simulink model "model"  (R2021b)
settings: Solver=VariableStepAuto  StartTime=0.0  StopTime=10.0  RelTol=1e-3
undefined symbols (not defined in the file): DiscIntNeverNeededParam
libraries: simulink x3, slpidlib x2
settings Model: Creator=O  LastModifiedBy=wangzixuan

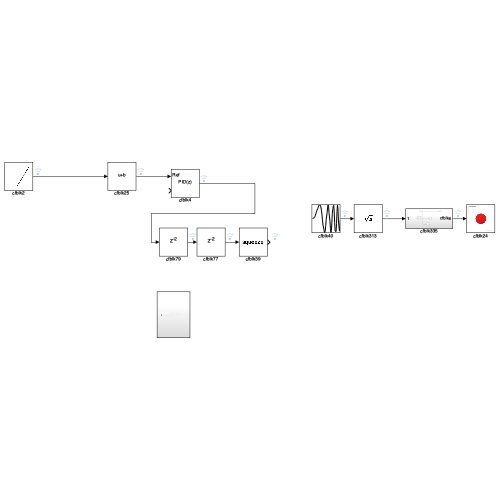
[thumbnail: Simulink's stored preview of the top-level diagram]
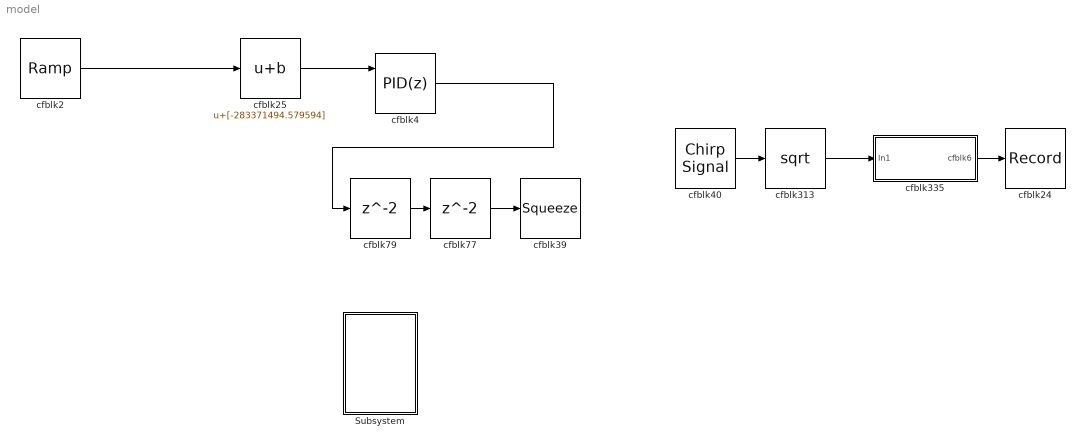
== system model ==
  Subsystem : Subsystem
  cfblk2 : simulink/Sources/Ramp  slope=[3073.754164]  start=[6.066803]  InitialOutput=[561595.891675]
  cfblk24 : Record  FileSettingsInternal="{\"entries\":[{\"content\":{\"excelSettings\":{\"content\":{},\"type\":\"Streamout.ExcelSettings\"}},\"type\":\"Streamout.FileSettingStorage\",\"uuid\":\"9c569ba5-3f76-45be-a7ff-ea8434ca4ceb\"}],\"packageUris\":[\"http://schema.mathworks.com/mf0/streamout_blocks/R2020a\"],\"version\":\"1.0\"}"  SignalsInternal="{\"entries\":[{\"content\":{\"signals\":[{\"content\":{\"blockPath\":[\"model/cfblk24\"],\"channel\":[],\"dimensions\":[1],\"domain\":\"model/cfblk24\",\"lineColor\":\"#ff13a6\",\"plots\":[1],\"port\":1,\"sid\":[],\"signalID\":585911,\"signalName\":\"cfblk335\"},\"type\":\"RecordBlkView.Signal\",\"uuid\":\"b2ada7c7-cfb3-4a8e-b65c-6ed73041aef6\"}]},\"type\":\"RecordBlkView.InputSignals\",\"uuid\":\"04f6ddc4-06cc-4646-89bd-e82fc14adc66\"}],\"packageUris\":[\"http://schema.mathworks.com/mf0/streamout_blocks/R2020a\"],\"version\":\"1.0\"}"  VisualizationBindings="{\"sparklinesplugin\":{\"info\":[{\"bindingParametersList\":[],\"subplotID\":1}]}}"
  cfblk25 : Bias  Bias=[-283371494.579594]
  cfblk313 : Sqrt  OutDataTypeStr=double  SaturateOnIntegerOverflow=on
  cfblk335 : Subsystem
  cfblk39 : Squeeze
  cfblk4 : slpidlib/PID Controller (2DOF)  Controller=PID  Form=Parallel  TimeDomain=Discrete-time  UseExternalTs=off  SampleTime=1  IntegratorMethod=Forward Euler  FilterMethod=Forward Euler  ControllerParametersSource=internal  P=1  I=1  D=0  UseFilter=on  N=100  b=1  c=1  TunerSelectOption=Transfer Function Based (PID Tuner App)  InitialConditionSource=internal  InitialConditionForIntegrator=0  InitialConditionForFilter=0  DifferentiatorICPrevScaledInput=0  ExternalReset=none  TrackingMode=off  Kt=1  LimitOutput=off  SatLimitsSource=internal  UpperSaturationLimit=inf  LowerSaturationLimit=-inf  LinearizeAsGain=off  AntiWindupMode=none  Kb=1  POutMin=[]  POutMax=[]  IOutMin=[]  IOutMax=[]  DOutMin=[]  DOutMax=[]  NOutMin=[]  NOutMax=[]  bOutMin=[]  bOutMax=[]  cOutMin=[]  cOutMax=[]  SumOutMin=[]  SumOutMax=[]  SaturationOutMin=[]  SaturationOutMax=[]  PParamMin=[]  PParamMax=[]  IParamMin=[]  IParamMax=[]  DParamMin=[]  DParamMax=[]  NParamMin=[]  NParamMax=[]  bParamMin=[]  bParamMax=[]  cParamMin=[]  cParamMax=[]  KbParamMin=[]  KbParamMax=[]  KtParamMin=[]  KtParamMax=[]  KbOutMin=[]  KbOutMax=[]  KtOutMin=[]  KtOutMax=[]  IntegratorOutMin=[]  IntegratorOutMax=[]  FilterOutMin=[]  FilterOutMax=[]  SumI1OutMin=[]  SumI1OutMax=[]  SumI2OutMin=[]  SumI2OutMax=[]  SumI3OutMin=[]  SumI3OutMax=[]  SumI4OutMin=[]  SumI4OutMax=[]  SumDOutMin=[]  SumDOutMax=[]  Sum1OutMin=[]  Sum1OutMax=[]  Sum2OutMin=[]  Sum2OutMax=[]  Sum3OutMin=[]  Sum3OutMax=[]  DifferentiatorOutMin=[]  DifferentiatorOutMax=[]  FilterDiffOutCoefMin=[]  FilterDiffOutCoefMax=[]  ReciprocalOutMin=[]  ReciprocalOutMax=[]  SumDenOutMin=[]  SumDenOutMax=[]  SumNumOutMin=[]  SumNumOutMax=[]  DivideOutMin=[]  DivideOutMax=[]  UdiffTsProdOutMin=[]  UdiffTsProdOutMax=[]  NTsProdOutMin=[]  NTsProdOutMax=[]  UintegralTsProdOutMin=[]  UintegralTsProdOutMax=[]  UngainTsProdOutMin=[]  UngainTsProdOutMax=[]  IntegratorContinuousStateAttributes=''  IntegratorStateMustResolveToSignalObject=off  IntegratorRTWStateStorageClass=Auto  FilterContinuousStateAttributes=''  FilterStateMustResolveToSignalObject=off  FilterRTWStateStorageClass=Auto  ParallelPVariant=InternalParameters  IdealPVariant=Disabled  IVariant=InternalParameters  DVariant=InternalParameters  bVariant=InternalParameters  cVariant=InternalParameters  IntegratorVariant=Discrete  SatVariant=Disabled  AWVariant=Passthrough  PCopyVariant=Disabled  TRVariant=Disabled  FdbkBlocksVariant=Forward  IdealPFdbkVariant=Disabled  SatFdbkVariant=Disabled  DerivativeFilterVariant=ForwardEulerFilter  NVariant=InternalParameters  NCopyVariant=Disabled  FilterICVariant=InternalICsFilter  IntegratorICVariant=InternalICs  ExternalResetVariant=Disabled  TRSumVariant=Passthrough  SumFdbkVariant=Disabled  SumVariant=Sum_PID  TsampFilterVariant=InternalTs  TsampNgainVariant=Passthrough  TsampIntegralVariant=Passthrough  ExternalSaturationOutDataTypeStr=Inherit: Same as second input
      settings: SourceProductBaseCode=SL
  cfblk40 : simulink/Sources/Chirp Signal  f1=[890112838.698821]  T=[783698053.297768]  f2=[819425252.339437]
  cfblk77 : Delay  SampleTime=1
  cfblk79 : Delay  SampleTime=1
  wires:
  cfblk335/1(cfblk6) -> cfblk24/1
  cfblk313/1 -> cfblk335/1(In1)
  cfblk40/1 -> cfblk313/1
  cfblk77/1 -> cfblk39/1
  cfblk2/1 -> cfblk25/1
  cfblk79/1 -> cfblk77/1
  cfblk4/1 -> cfblk79/1
  cfblk25/1 -> cfblk4/1

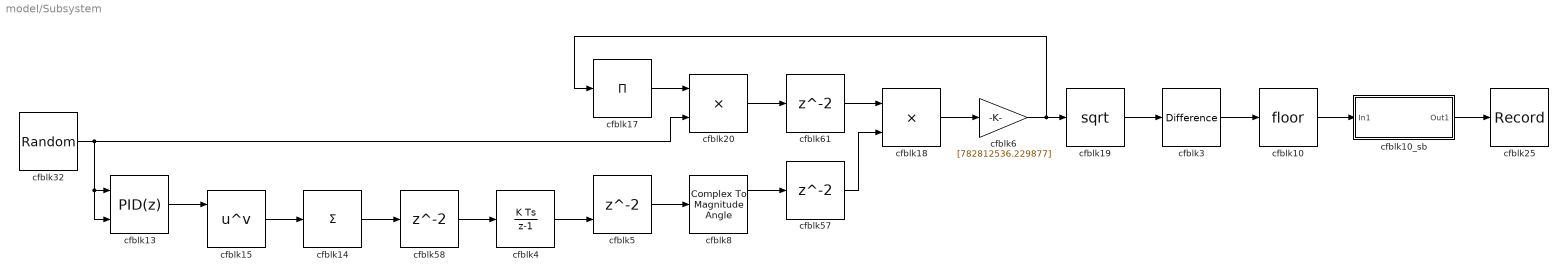
== system model/Subsystem ==
  cfblk10 : Rounding
  cfblk10_sb : Subsystem
  cfblk13 : slpidlib/PID Controller (2DOF)  Controller=PID  Form=Parallel  TimeDomain=Discrete-time  UseExternalTs=off  SampleTime=1  IntegratorMethod=Forward Euler  FilterMethod=Forward Euler  ControllerParametersSource=internal  P=1  I=1  D=0  UseFilter=on  N=100  b=1  c=1  TunerSelectOption=Transfer Function Based (PID Tuner App)  InitialConditionSource=internal  InitialConditionForIntegrator=0  InitialConditionForFilter=0  DifferentiatorICPrevScaledInput=0  ExternalReset=none  TrackingMode=off  Kt=1  LimitOutput=off  SatLimitsSource=internal  UpperSaturationLimit=inf  LowerSaturationLimit=-inf  LinearizeAsGain=off  AntiWindupMode=none  Kb=1  POutMin=[]  POutMax=[]  IOutMin=[]  IOutMax=[]  DOutMin=[]  DOutMax=[]  NOutMin=[]  NOutMax=[]  bOutMin=[]  bOutMax=[]  cOutMin=[]  cOutMax=[]  SumOutMin=[]  SumOutMax=[]  SaturationOutMin=[]  SaturationOutMax=[]  PParamMin=[]  PParamMax=[]  IParamMin=[]  IParamMax=[]  DParamMin=[]  DParamMax=[]  NParamMin=[]  NParamMax=[]  bParamMin=[]  bParamMax=[]  cParamMin=[]  cParamMax=[]  KbParamMin=[]  KbParamMax=[]  KtParamMin=[]  KtParamMax=[]  KbOutMin=[]  KbOutMax=[]  KtOutMin=[]  KtOutMax=[]  IntegratorOutMin=[]  IntegratorOutMax=[]  FilterOutMin=[]  FilterOutMax=[]  SumI1OutMin=[]  SumI1OutMax=[]  SumI2OutMin=[]  SumI2OutMax=[]  SumI3OutMin=[]  SumI3OutMax=[]  SumI4OutMin=[]  SumI4OutMax=[]  SumDOutMin=[]  SumDOutMax=[]  Sum1OutMin=[]  Sum1OutMax=[]  Sum2OutMin=[]  Sum2OutMax=[]  Sum3OutMin=[]  Sum3OutMax=[]  DifferentiatorOutMin=[]  DifferentiatorOutMax=[]  FilterDiffOutCoefMin=[]  FilterDiffOutCoefMax=[]  ReciprocalOutMin=[]  ReciprocalOutMax=[]  SumDenOutMin=[]  SumDenOutMax=[]  SumNumOutMin=[]  SumNumOutMax=[]  DivideOutMin=[]  DivideOutMax=[]  UdiffTsProdOutMin=[]  UdiffTsProdOutMax=[]  NTsProdOutMin=[]  NTsProdOutMax=[]  UintegralTsProdOutMin=[]  UintegralTsProdOutMax=[]  UngainTsProdOutMin=[]  UngainTsProdOutMax=[]  IntegratorContinuousStateAttributes=''  IntegratorStateMustResolveToSignalObject=off  IntegratorRTWStateStorageClass=Auto  FilterContinuousStateAttributes=''  FilterStateMustResolveToSignalObject=off  FilterRTWStateStorageClass=Auto  ParallelPVariant=InternalParameters  IdealPVariant=Disabled  IVariant=InternalParameters  DVariant=InternalParameters  bVariant=InternalParameters  cVariant=InternalParameters  IntegratorVariant=Discrete  SatVariant=Disabled  AWVariant=Passthrough  PCopyVariant=Disabled  TRVariant=Disabled  FdbkBlocksVariant=Forward  IdealPFdbkVariant=Disabled  SatFdbkVariant=Disabled  DerivativeFilterVariant=ForwardEulerFilter  NVariant=InternalParameters  NCopyVariant=Disabled  FilterICVariant=InternalICsFilter  IntegratorICVariant=InternalICs  ExternalResetVariant=Disabled  TRSumVariant=Passthrough  SumFdbkVariant=Disabled  SumVariant=Sum_PID  TsampFilterVariant=InternalTs  TsampNgainVariant=Passthrough  TsampIntegralVariant=Passthrough  ExternalSaturationOutDataTypeStr=Inherit: Same as second input
      settings: SourceProductBaseCode=SL
  cfblk14 : Sum  Inputs=+  OutDataTypeStr=double
  cfblk15 : Math  Operator=pow  OutDataTypeStr=double  SaturateOnIntegerOverflow=on
  cfblk17 : Product  Inputs=*  OutDataTypeStr=double
  cfblk18 : Product  Inputs=**  OutDataTypeStr=double
  cfblk19 : Sqrt  OutDataTypeStr=double  SaturateOnIntegerOverflow=on
  cfblk20 : Product  Inputs=**  OutDataTypeStr=double
  cfblk25 : Record  FileSettingsInternal="{\"entries\":[{\"content\":{\"excelSettings\":{\"content\":{},\"type\":\"Streamout.ExcelSettings\"}},\"type\":\"Streamout.FileSettingStorage\",\"uuid\":\"7687e2ec-381f-4673-acb7-97b648be0800\"}],\"packageUris\":[\"http://schema.mathworks.com/mf0/streamout_blocks/R2020a\"],\"version\":\"1.0\"}"  SignalsInternal="{\"entries\":[{\"content\":{\"signals\":[{\"content\":{\"blockPath\":[\"model/Subsystem/cfblk25\"],\"channel\":[],\"dimensions\":[1],\"domain\":\"model/Subsystem/cfblk25\",\"lineColor\":\"#d95319\",\"plots\":[1],\"port\":1,\"sid\":[],\"signalID\":585916,\"signalName\":\"cfblk10_sb\"},\"type\":\"RecordBlkView.Signal\",\"uuid\":\"a16bbc3b-36d9-44fd-905f-6b673a140423\"}]},\"type\":\"RecordBlkView.InputSignals\",\"uuid\":\"f5bc2cff-cab3-458f-b6f2-1f37294e6b90\"}],\"packageUris\":[\"http://schema.mathworks.com/mf0/streamout_blocks/R2020a\"],\"version\":\"1.0\"}"  VisualizationBindings="{\"sparklinesplugin\":{\"info\":[{\"bindingParametersList\":[],\"subplotID\":1}]}}"
  cfblk3 : simulink/Discrete/Difference  ICPrevInput=0.0  OutMin=[]  OutMax=[]  OutDataTypeStr=double  OutputDataTypeScalingMode=double  OutDataType=fixdt(1, 16)  OutScaling=2^-10  DoSatur=off
  cfblk32 : RandomNumber  Mean=[-73598.078492]  Variance=[73248.164035]  Seed=[877060262.000000]  SampleTime=0.1
  cfblk4 : DiscreteIntegrator  OutDataTypeStr=double  ICPrevOutput=DiscIntNeverNeededParam  ICPrevScaledInput=DiscIntNeverNeededParam
  cfblk5 : Delay  ShowEnablePort=on  SampleTime=1
      settings: InputPortMap=u0,e6
  cfblk57 : Delay  SampleTime=1
  cfblk58 : Delay  SampleTime=1
  cfblk6 : Gain  Gain=[782812536.229877]  OutDataTypeStr=double
  cfblk61 : Delay  SampleTime=1
  cfblk8 : ComplexToMagnitudeAngle
  wires:
  cfblk19/1 -> cfblk3/1
  cfblk57/1 -> cfblk18/2
  cfblk14/1 -> cfblk58/1
  cfblk6/1 -> cfblk19/1, cfblk17/1
  cfblk10_sb/1(Out1) -> cfblk25/1
  cfblk13/1 -> cfblk15/1
  cfblk18/1 -> cfblk6/1
  cfblk15/1 -> cfblk14/1
  cfblk20/1 -> cfblk61/1
  cfblk3/1 -> cfblk10/1
  cfblk58/1 -> cfblk4/1
  cfblk5/1 -> cfblk8/1
  cfblk10/1 -> cfblk10_sb/1(In1)
  cfblk61/1 -> cfblk18/1
  cfblk17/1 -> cfblk20/1
  cfblk4/1 -> cfblk5/2
  cfblk8/1 -> cfblk57/1
  cfblk32/1 -> cfblk13/2, cfblk13/1, cfblk20/2

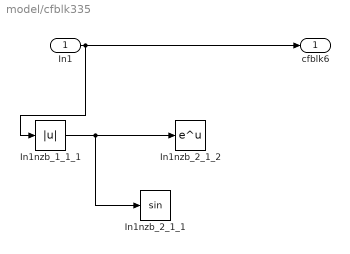
== system model/cfblk335 ==
  In1 : Inport
  In1nzb_1_1_1 : Abs
  In1nzb_2_1_1 : Trigonometry
  In1nzb_2_1_2 : Math  SaturateOnIntegerOverflow=on
  cfblk6 : Outport
  wires:
  In1/1 -> cfblk6/1, In1nzb_1_1_1/1
  In1nzb_1_1_1/1 -> In1nzb_2_1_1/1, In1nzb_2_1_2/1

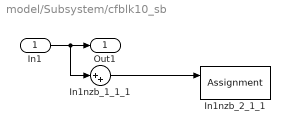
== system model/Subsystem/cfblk10_sb ==
  In1 : Inport
  In1nzb_1_1_1 : Sum  Inputs=|++
  In1nzb_2_1_1 : Assignment  DiagnosticForDimensions=Warning  IndexOptions=Index vector (dialog)  Indices=1  OutputSizes=1
  Out1 : Outport
  wires:
  In1/1 -> Out1/1, In1nzb_1_1_1/1
  In1nzb_1_1_1/1 -> In1nzb_2_1_1/1
